simulink model "States4"  (R2020a)
settings: Solver=FixedStepDiscrete  StartTime=0.0  StopTime=0.3  FixedStep=0.1  RelTol=1e-3  EnableMultiTasking=on
settings Model: Creator=bzhan  LastModifiedBy=bzhan
settings SolverCC: AutoInsertRateTranBlk=on
settings DataIOCC: LimitDataPoints=on
settings OptimizationCC: LifeSpan=inf
settings DebuggingCC: AllowSymbolicDim=off  SFUnexpectedBacktrackingDiag=warning  SFNoUnconditionalDefaultTransitionDiag=warning  SFExecutionAtInitializationDiag=none  ArithmeticOperatorsInVariantConditions=warning
settings SFSimCC: SimUseLocalCustomCode=off  CustomCodeUndefinedFunction=UseInterfaceOnly
settings RTWCC: RTWUseLocalCustomCode=off
settings CodeAppCC: StateflowObjectComments=on
settings GRTTargetCC: TargetLangStandard=C89/C90 (ANSI)
settings ConfigComp: CovMetricSettings=dw  CovHtmlReporting=on  CovSaveCumulativeToWorkspaceVar=on  CovSaveSingleToWorkspaceVar=on  CovShowResultsExplorer=off  CovExternalEMLEnable=off  CovSFcnEnable=off

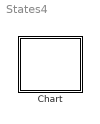
== system States4 ==
  Chart : Stateflow chart  TreatAsAtomicUnit=on

== stateflow chart States4/Chart ==
  settings: updateMethod=DISCRETE  sampleTime=0.1
  state A
    en: f("enA")
    du: f("duA")
    state A1
      en: f("enA1")
    state A2
      en: f("enA2")
    (default) -> A1
    A1 -> A2
  state B
    en: f("enB")
    du: f("duB")
    state B2
      en: f("enB2")
    state B1
      en: f("enB1")
    (default) -> B1
    B1 -> B2
  (default) -> A : {x=1;}
  B -> A : [x==2]{x=1;}
  A -> B : [x==1]{x=2;}
  data: s function_input; x local
  function f(s):
    | function f(s)
    |   fprintf(s+"\n");
